simulink model "up_counter"  (R2021a)
settings: Solver=VariableStepAuto  StartTime=0.0  StopTime=10.0  RelTol=1e-3
settings Model: Creator=DELL  LastModifiedBy=DELL

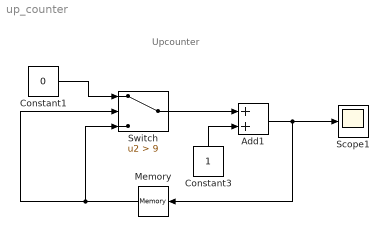
== system up_counter ==
  note: Upcounter
  Add1 : Sum
  Constant1 : Constant  Value=0
  Constant3 : Constant
  Memory : Memory
  Scope1 : Scope
  Switch : Switch  Criteria=u2 > Threshold  Threshold=9
  wires:
  Switch/1 -> Add1/1
  Constant3/1 -> Add1/2
  Memory/1 -> Switch/2, Switch/3
  Add1/1 -> Scope1/1, Memory/1
  Constant1/1 -> Switch/1
